simulink library "Lib_General_2016b"  (R2016b)
settings: Solver=VariableStepAuto  StartTime=0.0  StopTime=10.0  RelTol=1e-3
settings Model: Creator=62555  LastModifiedBy=62555
settings DataIOCC: ReturnWorkspaceOutputs=on
settings DebuggingCC: UnconnectedInputMsg=none  UnconnectedOutputMsg=none  UnconnectedLineMsg=none
settings ModelReferenceCC: EnableRefExpFcnMdlSchedulingChecks=off
settings SFSimCC: SimUseLocalCustomCode=on
settings RTWCC: RTWUseLocalCustomCode=on

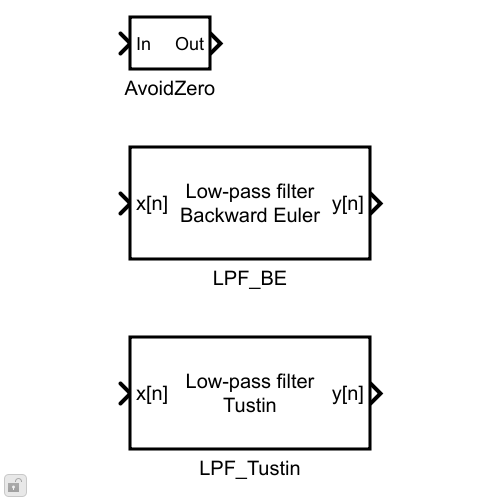
[thumbnail: Simulink's stored preview of the top-level diagram]
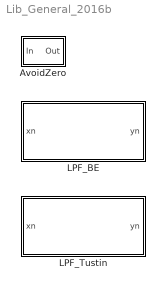
== system Lib_General_2016b ==
  AvoidZero : Subsystem  TreatAsAtomicUnit=on  RTWFileName=Lib_General
      settings: RTWFcnNameOpts=Use subsystem name  RTWFileNameOpts=User specified
  LPF_BE : Subsystem  TreatAsAtomicUnit=on  RTWFileName=Lib_PMSMCtrl  mask{tau=0, Ts=1, Initial_condition=0}
      settings: RTWFcnNameOpts=Use subsystem name  RTWFileNameOpts=User specified
      mask Display:
      | disp('Low-pass filter\nBackward Euler');
      | port_label('input', 1, 'x[n]');
      | port_label('output', 1, 'y[n]');
  LPF_Tustin : Subsystem  TreatAsAtomicUnit=on  RTWFileName=Lib_PMSMCtrl  mask{tau=0, Ts=1, Initial_condition=0}
      settings: RTWFcnNameOpts=Use subsystem name  RTWFileNameOpts=User specified
      mask Display:
      | disp('Low-pass filter\nTustin');
      | port_label('input', 1, 'x[n]');
      | port_label('output', 1, 'y[n]');

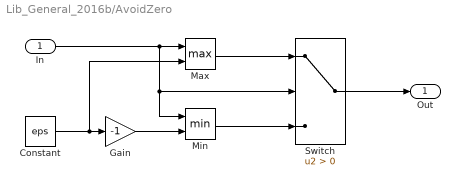
== system Lib_General_2016b/AvoidZero ==
  In : Inport
  Constant : Constant  Value=eps  OutDataTypeStr=single  SampleTime=-1
  Gain : Gain  Gain=-1
  Max : MinMax  Function=max  Inputs=2
  Min : MinMax  Inputs=2
  Switch : Switch  Criteria=u2 > Threshold
  Out : Outport
  wires:
  In/1 -> Min/1, Switch/2, Max/1
  Max/1 -> Switch/1
  Gain/1 -> Min/2
  Min/1 -> Switch/3
  Constant/1 -> Max/2, Gain/1
  Switch/1 -> Out/1

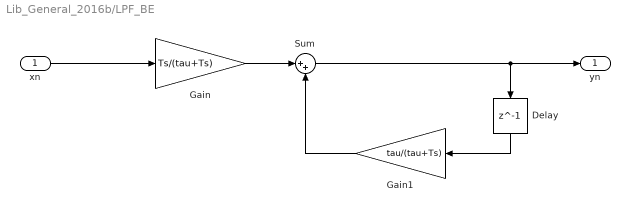
== system Lib_General_2016b/LPF_BE ==
  xn : Inport
  Delay : Delay  DelayLength=1  InitialCondition=Initial_condition
  Gain : Gain  Gain=Ts/(tau+Ts)
  Gain1 : Gain  Gain=tau/(tau+Ts)
  Sum : Sum  Inputs=|++
  yn : Outport
  wires:
  Delay/1 -> Gain1/1
  xn/1 -> Gain/1
  Gain/1 -> Sum/1
  Sum/1 -> yn/1, Delay/1
  Gain1/1 -> Sum/2

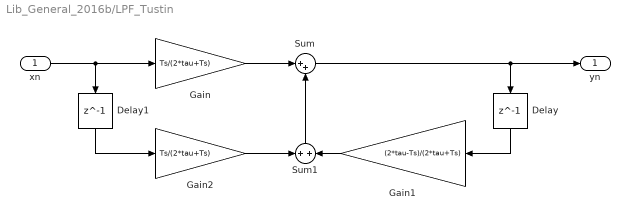
== system Lib_General_2016b/LPF_Tustin ==
  xn : Inport
  Delay : Delay  DelayLength=1  InitialCondition=Initial_condition
  Delay1 : Delay  DelayLength=1  InitialCondition=Initial_condition
  Gain : Gain  Gain=Ts/(2*tau+Ts)
  Gain1 : Gain  Gain=(2*tau-Ts)/(2*tau+Ts)
  Gain2 : Gain  Gain=Ts/(2*tau+Ts)
  Sum : Sum  Inputs=|++
  Sum1 : Sum  Inputs=+|+
  yn : Outport
  wires:
  Delay/1 -> Gain1/1
  xn/1 -> Gain/1, Delay1/1
  Gain/1 -> Sum/1
  Sum/1 -> yn/1, Delay/1
  Gain1/1 -> Sum1/2
  Gain2/1 -> Sum1/1
  Sum1/1 -> Sum/2
  Delay1/1 -> Gain2/1
